simulink model "Bioreactor"  (R2014b)
settings: Solver=ode45  StartTime=0.0  StopTime=100  MaxStep=0.5  RelTol=1e-3
settings Model: Creator=jeff  LastModifiedBy=jeff
settings DataIOCC: ExternalInput=[t,u]

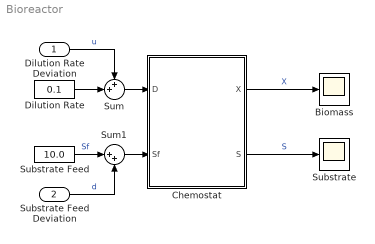
== system Bioreactor ==
  Dilution Rate Deviation : Inport
  Substrate Feed Deviation : Inport  Port=2
  Biomass : Scope
      settings: TimeRange=100  YMin=0
  Chemostat : Subsystem
      mask Display: image(imread('Bioreactor_schematic.png'))
  Dilution Rate : Constant  Value=0.1
  Substrate : Scope
      settings: TimeRange=100  YMin=0  YMax=10
  "Substrate Feed " : Constant  Value=10.0
  Sum : Sum  Inputs=++|
  Sum1 : Sum  Inputs=|++
  wires:
  Chemostat/1(X) -> Biomass/1  "X"
  Chemostat/2(S) -> Substrate/1  "S"
  Sum/1 -> Chemostat/1(D)
  Dilution Rate/1 -> Sum/2
  Dilution Rate Deviation/1 -> Sum/1  "u"
  Sum1/1 -> Chemostat/2(Sf)
  "Substrate Feed "/1 -> Sum1/1  "Sf"
  Substrate Feed Deviation/1 -> Sum1/2  "d"

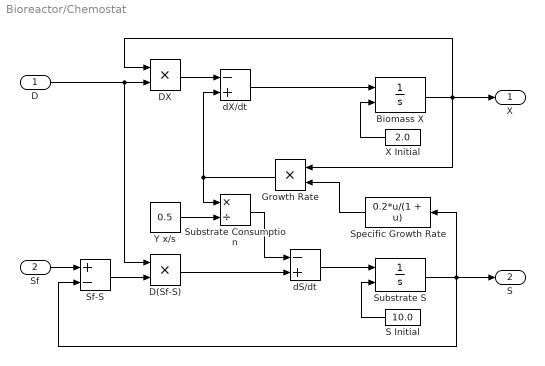
== system Bioreactor/Chemostat ==
  D : Inport
  Sf : Inport  Port=2
  Biomass X : Integrator  InitialConditionSource=external  InitialCondition=0.5  LimitOutput=on  UpperSaturationLimit=Inf  LowerSaturationLimit=0  ContinuousStateAttributes='biomass'
  D(Sf-S) : Product
  DX : Product
  Growth Rate : Product
  S Initial : Constant  Value=10.0
  Sf-S : Sum  Inputs=+-
  Specific Growth Rate : Fcn  Expr=0.2*u/(1 + u)
  Substrate Consumption : Product  Inputs=*/
  Substrate S : Integrator  InitialConditionSource=external  InitialCondition=0.0  LimitOutput=on  UpperSaturationLimit=Inf  LowerSaturationLimit=0  ContinuousStateAttributes='substrate'
  X Initial : Constant  Value=2.0
  Y x/s : Constant  Value=0.5
  dS/dt : Sum  Inputs=-+
  dX/dt : Sum  Inputs=-+
  X : Outport
  S : Outport  Port=2
  wires:
  Biomass X/1 -> Growth Rate/1, X/1, DX/1
  DX/1 -> dX/dt/1
  dS/dt/1 -> Substrate S/1
  Substrate Consumption/1 -> dS/dt/1
  Y x/s/1 -> Substrate Consumption/2
  Sf-S/1 -> D(Sf-S)/2
  Specific Growth Rate/1 -> Growth Rate/2
  dX/dt/1 -> Biomass X/1
  D/1 -> D(Sf-S)/1, DX/2
  D(Sf-S)/1 -> dS/dt/2
  Substrate S/1 -> Specific Growth Rate/1, S/1, Sf-S/2
  Growth Rate/1 -> Substrate Consumption/1, dX/dt/2
  Sf/1 -> Sf-S/1
  X Initial/1 -> Biomass X/2
  S Initial/1 -> Substrate S/2
